simulink model "ComputedTorqueControl"  (R2019b)
settings: Solver=ode23t  StartTime=0.0  StopTime=20  FixedStep=0.01  MaxStep=0.05  RelTol=1e-3  EnableMultiTasking=on
PreLoadFcn:
  | mdl_puma560
values from neighbouring files (symbols this model uses):
  R = SerialLink(L, 'name', '210F', 'comment', 'six DOF', 'manufacturer', 'FANUC')    [Model_210F.m]    (also in Model_210F_old.m)
undefined symbols (not defined in the file or in its folder): slcoulomb
libraries: roblocks x12, simulink x1
settings Model: ExtModeTrigMode=oneshot  ExtModeArmWhenConnect=off  Creator=pic  LastModifiedBy=Karl
settings SolverCC: ZeroCrossControl=DisableAll
settings DataIOCC: SaveFormat=Array  SignalLoggingSaveFormat=ModelDataLogs  TimeSaveName=t  OutputSaveName=y  ReturnWorkspaceOutputsName=Rsim
settings OptimizationCC: BlockReduction=off  BooleanDataType=off  ExpressionDepthLimit=2147483647  InitFltsAndDblsToZero=on  LifeSpan=inf
settings DebuggingCC: SaveWithParameterizedLinksMsg=none  UnderspecifiedInitializationDetection=Classic  MergeDetectMultiDrivingBlocksExec=none  SignalResolutionControl=TryResolveAllWithWarning  MultiTaskDSMMsg=warning  MultiTaskCondExecSysMsg=none  FcnCallInpInsideContextMsg=warning  AllowSymbolicDim=off  StateNameClashWarn=warning  SFUnexpectedBacktrackingDiag=warning  SFNoUnconditionalDefaultTransitionDiag=warning  SFExecutionAtInitializationDiag=none  ArithmeticOperatorsInVariantConditions=warning
settings HardwareCC: ProdBitPerPointer=32  ProdBitPerSizeT=32  ProdBitPerPtrDiffT=32  ProdLargestAtomicFloat=None  ProdIntDivRoundTo=Undefined  ProdEndianess=Unspecified  ProdWordSize=32  ProdHWDeviceType=32-bit Generic  TargetUnknown=on
settings ModelReferenceCC: PropagateSignalLabelsOutOfModel=off
settings SFSimCC: SimUseLocalCustomCode=off  CustomCodeUndefinedFunction=UseInterfaceOnly
settings RTWCC: RTWUseLocalCustomCode=off
settings CodeAppCC: StateflowObjectComments=on
settings GRTTargetCC: TargetLangStandard=C89/C90 (ANSI)  ModelReferenceCompliant=off  CompOptLevelCompliant=off  GeneratePreprocessorConditionals=Disable all  CombineOutputUpdateFcns=off  MatFileLogging=off  GRTInterface=on
settings ConfigComp: CovMetricSettings=dw  CovHtmlReporting=on  CovSaveCumulativeToWorkspaceVar=on  CovSaveSingleToWorkspaceVar=on  CovExternalEMLEnable=off

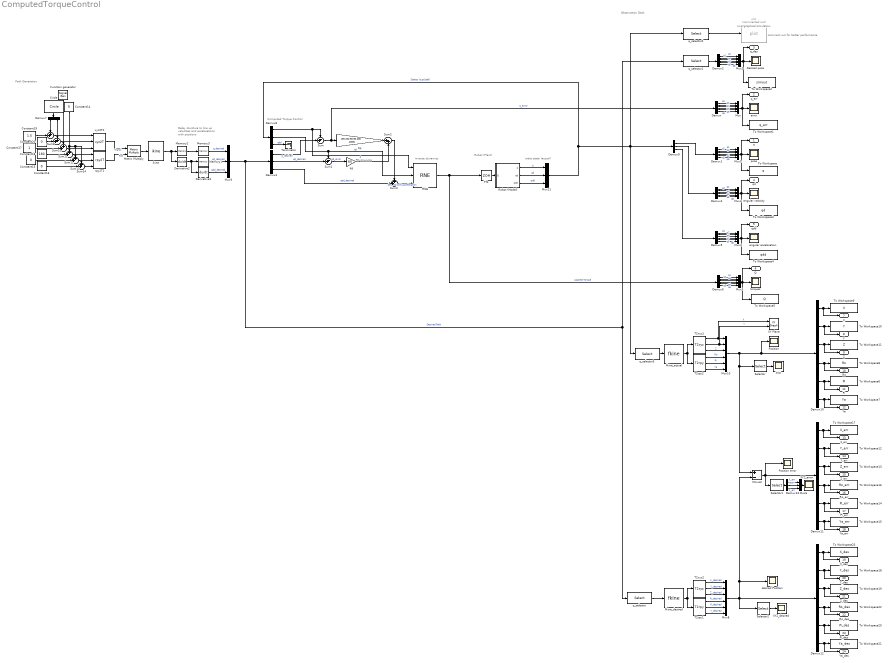
== system ComputedTorqueControl ==
  note: Observation Deck
  note: Robot (Plant)
  note: Path Generation
  note: inverse dynamics
  note: robot state
      | (actual)
  note: Computed Torque Control
  note: Delay sturcture to line up velocities and accelerations with positions
  note: PD-strucutre
  note: Live graphical simulation
  note: comment out for better performance
  "Circle " : roblocks/Toolbox/Circle  radius=0.5  freq=0.1
  Constant{14..16,20} (4 alike) : Constant  Value=0
  Constant17 : Constant
  Constant18 : Constant  Value=180
  Constant19 : Constant  Value=1.5
  Demux{,1..2,4..6,10..12} (9 alike) : Demux  Outputs=6
  Demux{3,8..9,13} (4 alike) : Demux  Outputs=3
  Demux7 : Demux  Outputs=2
  Derivative2 : Derivative
  Derivative3 : Derivative
  Desired pose : Scope
  Function generator : SignalGenerator  Amplitude=0.1  Frequency=0.2
  Kd : Gain  Gain=60  SaturateOnIntegerOverflow=on  OutDataTypeStr=Inherit: Same as input  ParamDataTypeStr=Inherit: Same as input
  Kp : Gain  Gain=[90 200 90 90 200 1000]  SaturateOnIntegerOverflow=on  OutDataTypeStr=Inherit: Same as input  ParamDataTypeStr=Inherit: Same as input
  Matrix Multiply : Product  Multiplication=Matrix(*)
  Memory1 : Memory  InitialCondition=[0 0 0 0 0 0]  InheritSampleTime=on
  Memory2 : Memory  InitialCondition=[0 0 0 0 0 0]  InheritSampleTime=on
  Memory3 : Memory  InitialCondition=[0 0 0 0 0 0]  InheritSampleTime=on
  Minus3 : Sum  Inputs=+-
  Mux{,1..5,8,10} (8 alike) : Mux  Inputs=6
  Mux11 : Mux  Inputs=3
  Mux6 : Mux  Inputs=3
  Mux9 : Mux  Inputs=3
  Position : Scope
  Position error : Scope
  RNE : roblocks/Arm/RNE  robot=R.nofriction  grav=[0 0 9.81]
  Robot (Model) : Subsystem  AncestorBlock=roblocks/Arm/Robot  mask{robot=R.nofriction, q0=[0 -pi/4 0 0 -pi/4 0]}
      mask prompts: robot "Robot object"; q0 "Initial state"
      mask help: Rigid-body dynamic model of robot.
      mask init:
      | if isa(robot, 'SerialLink')
      |     rname = robot.name;
      |     %fprintf('**robot name is %s\n', rname);
      | else
      |     rname = '';
      |     n = 0
      | end
      mask Help:
      | Simulates the forward (direct) rigid-body dynamics of the robot described
      | by the given robot object.  For given applied joint torque/force it computes
      | the instaneous joint coordinates, velocities and acclerations.
      | 
      | 
      | <b>Parameters::</b>
      | 
      | robot (SerialLink) a dynamic model of an N-link serial link manipulator
      | q0 (1xN)  Initial joint coordinates
      | 
      | <b>Inputs::</b>
      | 
      | Q (1xN) the generalized joint force (torque or force) required to achieve
      | the motion state (q, qd, qdd).
      | 
      | <b>Outputs::</b>
      | 
      | q (1xN) joint coordinates
      | qd (1xN) joint coordinate velocity
      | qdd (1xN) joint coordinate acceleration
      | 
      | 
      | <b>Notes::</b>
      | 
      | - Required to simulate robot rigid body motion.
      | - Implemented using the recursive Newton-Euler scheme (RNE).
      | - A wrapper for the Toolbox method accel() which in turn depends on the
      |   method rne().
      mask Display:
      | port_label('input', 1, 'Q')
      | port_label('output', 1, 'q')
      | port_label('output', 2, 'qd')
      | port_label('output', 3, 'qdd')
      | text(0.1, 0.9,  rname, 'horizontalAlignment', 'left')
  Selector : Selector  InputPortWidth=6  IndexOptions=Index vector (dialog)  Indices=[1 2 3]  OutputSizes=1
  Selector1 : Selector  InputPortWidth=6  IndexOptions=Index vector (dialog)  Indices=[1 2 3]  OutputSizes=1
  Selector2 : Selector  InputPortWidth=6  IndexOptions=Index vector (dialog)  Indices=[1 2 3]  OutputSizes=1
  Sum : Sum  Inputs=-+|  SaturateOnIntegerOverflow=on  InputSameDT=on  OutDataTypeStr=Inherit: Same as first input
  Sum1 : Sum  Inputs=-+|  SaturateOnIntegerOverflow=on  InputSameDT=on  OutDataTypeStr=Inherit: Same as first input
  Sum{8,10..14} (6 alike) : Sum  Inputs=++|
  Sum2 : Sum  Inputs=|++  SaturateOnIntegerOverflow=on  InputSameDT=on  OutDataTypeStr=Inherit: Same as first input
  Sum3 : Sum  Inputs=++|  SaturateOnIntegerOverflow=on  InputSameDT=on  OutDataTypeStr=Inherit: Same as first input
  T2rpy1 : roblocks/Toolbox/T2rpy  sequence=ZYX  degrees=off
  T2rpy2 : roblocks/Toolbox/T2rpy  sequence=ZYX  degrees=off
  T2xyz1 : roblocks/Toolbox/T2xyz
  T2xyz2 : roblocks/Toolbox/T2xyz
  Terminator : Terminator
  Tfb : ZeroOrderHold  SampleTime=0.005
  To Workspace : ToWorkspace  VariableName=q  SaveFormat=Timeseries  SampleTime=-1
  To Workspace1 : ToWorkspace  VariableName=q_err  SaveFormat=Timeseries  SampleTime=-1
  To Workspace10 : ToWorkspace  VariableName=Y  SaveFormat=Timeseries  SampleTime=-1
  To Workspace11 : ToWorkspace  VariableName=Z  SaveFormat=Timeseries  SampleTime=-1
  To Workspace12 : ToWorkspace  VariableName=Y_err  SaveFormat=Timeseries  SampleTime=-1
  To Workspace13 : ToWorkspace  VariableName=Z_err  SaveFormat=Timeseries  SampleTime=-1
  To Workspace14 : ToWorkspace  VariableName=Pi_err  SaveFormat=Timeseries  SampleTime=-1
  To Workspace15 : ToWorkspace  VariableName=Ya_err  SaveFormat=Timeseries  SampleTime=-1
  To Workspace16 : ToWorkspace  VariableName=Ro_err  SaveFormat=Timeseries  SampleTime=-1
  To Workspace17 : ToWorkspace  VariableName=X_err  SaveFormat=Timeseries  SampleTime=-1
  To Workspace18 : ToWorkspace  VariableName=Y_des  SaveFormat=Timeseries  SampleTime=-1
  To Workspace19 : ToWorkspace  VariableName=Z_des  SaveFormat=Timeseries  SampleTime=-1
  To Workspace2 : ToWorkspace  VariableName=simout  SaveFormat=Timeseries  SampleTime=-1
  To Workspace20 : ToWorkspace  VariableName=Pi_des  SaveFormat=Timeseries  SampleTime=-1
  To Workspace21 : ToWorkspace  VariableName=Ya_des  SaveFormat=Timeseries  SampleTime=-1
  To Workspace22 : ToWorkspace  VariableName=Ro_des  SaveFormat=Timeseries  SampleTime=-1
  To Workspace23 : ToWorkspace  VariableName=X_des  SaveFormat=Timeseries  SampleTime=-1
  To Workspace3 : ToWorkspace  VariableName=qd  SaveFormat=Timeseries  SampleTime=-1
  To Workspace4 : ToWorkspace  VariableName=qdd  SaveFormat=Timeseries  SampleTime=-1
  To Workspace5 : ToWorkspace  VariableName=Q  SaveFormat=Timeseries  SampleTime=-1
  To Workspace6 : ToWorkspace  VariableName=Pi  SaveFormat=Timeseries  SampleTime=-1
  To Workspace7 : ToWorkspace  VariableName=Ya  SaveFormat=Timeseries  SampleTime=-1
  To Workspace8 : ToWorkspace  VariableName=Ro  SaveFormat=Timeseries  SampleTime=-1
  To Workspace9 : ToWorkspace  VariableName=X  SaveFormat=Timeseries  SampleTime=-1
  XY Plane : simulink/Sinks/XY Graph  xmin=-3  xmax=3  ymin=-3  ymax=3  st=-1
  XYZ : Scope
  XYZ_desired : Scope
  XYZ_error : Scope
  angular acceleration : Scope
  angular velocity : Scope
  desired Position : Scope
  error : Scope
  fkine_actual : roblocks/Arm/fkine  robot=R.nofriction
  fkine_desired : roblocks/Arm/fkine  robot=R.nofriction
  ikine : roblocks/Arm/ikine  robot=R.nofriction  q0=[0 -pi/4 0 0 -pi/4 0]  M=[1 1 1 1 1 1]  pinv=off  options={}
  plot : roblocks/Arm/plot  Commented=on  robot=R.nofriction  fps=10  holdplot=on
  pose : Scope
  q_selector{,1..3} (4 alike) : Selector  InputPortWidth=18  IndexOptions=Index vector (dialog)  Indices=[1 2 3 4 5 6]  OutputSizes=1
  rpy2T2 : roblocks/Toolbox/rpy2T  sequence=ZYX  degrees=on
  torques : Scope
  xyz2T2 : roblocks/Toolbox/xyz2T
  q : Outport  VectorParamsAs1DForOutWhenUnconnected=off
  q_err : Outport  Port=2  VectorParamsAs1DForOutWhenUnconnected=off
  q_des : Outport  Port=3
  qd : Outport  Port=4  VectorParamsAs1DForOutWhenUnconnected=off
  qdd : Outport  Port=5  VectorParamsAs1DForOutWhenUnconnected=off
  Q : Outport  Port=6  VectorParamsAs1DForOutWhenUnconnected=off
  X : Outport  Port=7  VectorParamsAs1DForOutWhenUnconnected=off
  Y : Outport  Port=8  VectorParamsAs1DForOutWhenUnconnected=off
  Z : Outport  Port=9
  Ro : Outport  Port=10  VectorParamsAs1DForOutWhenUnconnected=off
  Pi : Outport  Port=11  VectorParamsAs1DForOutWhenUnconnected=off
  Ya : Outport  Port=12
  X_err : Outport  Port=13  VectorParamsAs1DForOutWhenUnconnected=off
  Y_err : Outport  Port=14  VectorParamsAs1DForOutWhenUnconnected=off
  Z_err : Outport  Port=15
  Ro_err : Outport  Port=16  VectorParamsAs1DForOutWhenUnconnected=off
  Pi_err : Outport  Port=17  VectorParamsAs1DForOutWhenUnconnected=off
  Ya_err : Outport  Port=18
  X_des : Outport  Port=19  VectorParamsAs1DForOutWhenUnconnected=off
  Y_des : Outport  Port=20  VectorParamsAs1DForOutWhenUnconnected=off
  Z_des : Outport  Port=21
  Ro_des : Outport  Port=22  VectorParamsAs1DForOutWhenUnconnected=off
  Pi_des : Outport  Port=23  VectorParamsAs1DForOutWhenUnconnected=off
  Ya_des : Outport  Port=24
  wires:
  Kp/1 -> Sum2/1
  Kd/1 -> Sum2/2
  Sum3/1 -> RNE/3  "desired joint acceleration"
  Sum2/1 -> Sum3/1
  Mux/1 -> q_err/1, To Workspace1/1, error/1
  Demux/4 -> Mux/4  "q4"
  Demux/5 -> Mux/5  "q5"
  Demux/6 -> Mux/6  "q6"
  Demux/3 -> Mux/3  "q3"
  Demux/2 -> Mux/2  "q2"
  Sum/1 -> Demux/1, Kp/1  "q_error"
  Demux/1 -> Mux/1  "q1"
  Mux1/1 -> q/1, To Workspace/1, pose/1
  Demux1/6 -> Mux1/6  "q6"
  Demux1/3 -> Mux1/3  "q3"
  Demux1/2 -> Mux1/2  "q2"
  Demux1/5 -> Mux1/5  "q5"
  Demux1/1 -> Mux1/1  "q1"
  Demux1/4 -> Mux1/4  "q4"
  Demux2/4 -> Mux2/4  "q4"
  Demux2/1 -> Mux2/1  "q1"
  Demux2/5 -> Mux2/5  "q5"
  Demux2/2 -> Mux2/2  "q2"
  Demux2/3 -> Mux2/3  "q3"
  Demux2/6 -> Mux2/6  "q6"
  Mux2/1 -> Desired pose/1, q_des/1, To Workspace2/1
  Demux4/1 -> Mux3/1  "q1"
  Mux3/1 -> qd/1, To Workspace3/1, angular velocity/1
  Demux4/5 -> Mux3/5  "q5"
  Demux4/2 -> Mux3/2  "q2"
  Demux4/6 -> Mux3/6  "q6"
  Demux4/4 -> Mux3/4  "q4"
  Demux4/3 -> Mux3/3  "q3"
  Demux5/2 -> Mux4/2  "q2"
  Demux5/5 -> Mux4/5  "q5"
  Demux5/6 -> Mux4/6  "q6"
  Robot (Model)/3(qdd) -> Mux11/3  "qdd"
  Mux4/1 -> qdd/1, To Workspace4/1, angular acceleration/1
  Demux5/1 -> Mux4/1  "q1"
  Demux5/4 -> Mux4/4  "q4"
  Demux5/3 -> Mux4/3  "q3"
  Sum1/1 -> Kd/1  "qd_error"
  Demux6/1 -> Mux5/1  "q1"
  Demux6/3 -> Mux5/3  "q3"
  Mux5/1 -> Q/1, To Workspace5/1, torques/1
  Demux6/6 -> Mux5/6  "q6"
  Demux6/2 -> Mux5/2  "q2"
  Demux6/4 -> Mux5/4  "q4"
  Demux6/5 -> Mux5/5  "q5"
  Robot (Model)/1(q) -> Mux11/1  "q"
  Tfb/1 -> Robot (Model)/1(Q)
  Memory2/1 -> Memory3/1
  ikine/1 -> Memory2/1, Derivative2/1
  RNE/1 -> Demux6/1, Tfb/1  "Applied Torque"
  Robot (Model)/2(qd) -> Mux11/2  "qd"
  T2rpy1/2 -> Mux8/5  "P_desired"
  T2rpy1/3 -> Mux8/6  "Y_desired"
  T2xyz2/3 -> Mux8/3  "Z_desired"
  T2xyz2/2 -> Mux8/2  "Y_desired"
  T2xyz2/1 -> Mux8/1  "X_desired"
  T2rpy1/1 -> Mux8/4  "R_desired"
  Matrix Multiply/1 -> ikine/1
  Sum8/1 -> xyz2T2/1
  xyz2T2/1 -> Matrix Multiply/1  "Transl"
  Constant14/1 -> Sum14/1, Sum13/1, Sum12/1
  Constant17/1 -> Sum11/2
  Demux7/1 -> Sum8/1
  Sum14/1 -> rpy2T2/3
  rpy2T2/1 -> Matrix Multiply/2  "Rot"
  Demux7/2 -> Sum10/1
  Sum12/1 -> rpy2T2/1
  Constant15/1 -> Sum13/2
  Constant16/1 -> Sum14/2
  Function generator/1 -> Sum11/1
  Sum11/1 -> xyz2T2/3
  Constant18/1 -> Sum12/2
  Constant20/1 -> Sum10/2
  Constant19/1 -> Sum8/2
  Sum13/1 -> rpy2T2/2
  Sum10/1 -> xyz2T2/2
  "Circle "/1 -> Demux7/1
  Derivative2/1 -> Memory1/1, Derivative3/1
  Memory3/1 -> Mux9/1  "q_desired"
  Memory1/1 -> Mux9/2  "qd_desired"
  Derivative3/1 -> Mux9/3  "qdd_desired"
  Demux3/1 -> Sum/2  "q_desired"
  Demux3/2 -> Sum1/2  "qd_desired"
  Demux3/3 -> Sum3/2  "qdd_desired"
  Mux9/1 -> Demux3/1, q_selector/1, q_selector1/1  "Desired Path"
  fkine_desired/1 -> T2xyz2/1, T2rpy1/1
  T2rpy2/3 -> Mux10/6  "Ya"
  T2rpy2/1 -> Mux10/4  "Ro"
  T2xyz1/2 -> XY Plane/2, Mux10/2  "Y"
  T2xyz1/3 -> Mux10/3  "Z"
  T2rpy2/2 -> Mux10/5  "Pi"
  T2xyz1/1 -> XY Plane/1, Mux10/1  "X"
  fkine_actual/1 -> T2rpy2/1, T2xyz1/1
  q_selector/1 -> fkine_desired/1
  Mux10/1 -> Position/1, Demux10/1, Selector/1, Minus3/1
  q_selector1/1 -> Demux2/1
  Mux11/1 -> Demux8/1, Demux9/1, q_selector2/1, q_selector3/1  "States (q,qd,qdd)"
  Demux8/1 -> RNE/1, Sum/1  "q"
  Demux8/2 -> Sum1/1, RNE/2  "qd"
  Demux8/3 -> Terminator/1  "qdd"
  Demux9/2 -> Demux4/1
  Demux9/3 -> Demux5/1
  Demux9/1 -> Demux1/1
  q_selector2/1 -> plot/1
  q_selector3/1 -> fkine_actual/1
  Demux10/1 -> To Workspace9/1, X/1
  Demux10/2 -> Y/1, To Workspace10/1
  Demux10/3 -> Z/1, To Workspace11/1
  Demux10/4 -> Ro/1, To Workspace8/1
  Demux10/5 -> Pi/1, To Workspace6/1
  Demux10/6 -> Ya/1, To Workspace7/1
  Demux11/6 -> Ya_err/1, To Workspace15/1
  Demux11/3 -> Z_err/1, To Workspace13/1
  Minus3/1 -> Demux11/1, Position error/1, Selector1/1
  Demux11/4 -> Ro_err/1, To Workspace16/1
  Demux11/2 -> Y_err/1, To Workspace12/1
  Demux11/5 -> Pi_err/1, To Workspace14/1
  Demux11/1 -> To Workspace17/1, X_err/1
  Demux12/6 -> Ya_des/1, To Workspace21/1
  Demux12/3 -> Z_des/1, To Workspace19/1
  Mux8/1 -> Demux12/1, Selector2/1, desired Position/1, Minus3/2
  Demux12/4 -> Ro_des/1, To Workspace22/1
  Demux12/2 -> Y_des/1, To Workspace18/1
  Demux12/5 -> Pi_des/1, To Workspace20/1
  Demux12/1 -> To Workspace23/1, X_des/1
  Selector/1 -> XYZ/1
  Selector1/1 -> Demux13/1
  Selector2/1 -> XYZ_desired/1
  Demux13/1 -> Mux6/1  "X_err"
  Demux13/2 -> Mux6/2  "Y_err"
  Demux13/3 -> Mux6/3  "Z_err"
  Mux6/1 -> XYZ_error/1

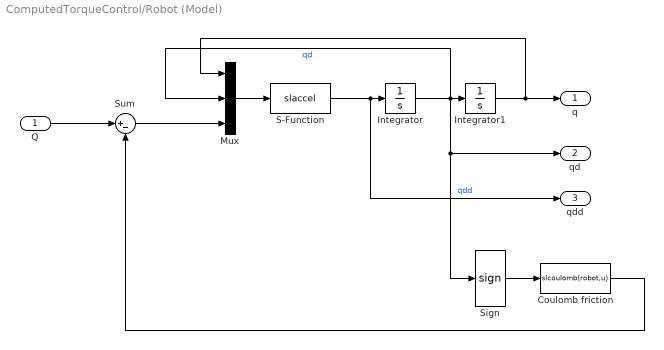
== system ComputedTorqueControl/Robot (Model) ==
  Q : Inport
  Coulomb friction : MATLABFcn  MATLABFcn=slcoulomb(robot,u)  OutputDimensions=[robot.n 1]  Output1D=off
  Integrator : Integrator
  Integrator1 : Integrator  InitialCondition=q0
  Mux : Mux  Inputs=3
  S-Function : S-Function  FunctionName=slaccel  Parameters=robot  SFunctionDeploymentMode=off  EnableBusSupport=off
  Sign : Signum
  Sum : Sum  Inputs=|+-
  q : Outport  VectorParamsAs1DForOutWhenUnconnected=off
  qd : Outport  Port=2  VectorParamsAs1DForOutWhenUnconnected=off
  qdd : Outport  Port=3  VectorParamsAs1DForOutWhenUnconnected=off
  wires:
  S-Function/1 -> qdd/1, Integrator/1  "qdd"
  Mux/1 -> S-Function/1
  Integrator/1 -> Sign/1, qd/1, Integrator1/1, Mux/2  "qd"
  Integrator1/1 -> q/1, Mux/1
  Q/1 -> Sum/1
  Sum/1 -> Mux/3
  Coulomb friction/1 -> Sum/2
  Sign/1 -> Coulomb friction/1
